simulink model "HVACRelay_harness"  (Simulink 7.7)
settings: Solver=FixedStepDiscrete  SolverMode=SingleTasking  StartTime=0.0  StopTime=100  FixedStep=.01  RelTol=1e-3
PostLoadFcn:
  | cd '..';
  | PostLoadFcn;
  | cd 'harness';
InitFcn:
  | if signalbuilder('HVACRelay_harness/Signal Builder','activegroup') == 1
  |   CD_HVAC_RELAY_FUNCTION.DataType = 'uint8';
  |   CD_HVAC_RELAY_FUNCTION.Value = 255;
  |   CD_HVAC_RELAY_FEEDBACK_FUNCTION.DataType = 'uint8';
  |   CD_HVAC_RELAY_FEEDBACK_FUNCTION.Value = 255;
  | else
  |   CD_HVAC_RELAY_FUNCTION.DataType = 'uint8';
  |   CD_HVAC_RELAY_FUNCTION.Value = 0;
  |   CD_HVAC_RELAY_FEEDBACK_FUNCTION.DataType = 'uint8';
  |   CD_HVAC_RELAY_FEEDBACK_FUNCTION.Value = 0;
  | end
undefined symbols (not defined in the file): ACTIVE, CD_HVAC_RELAY_DEBOUNCE_ERROR_ON, ENGINE_CRANKING, INACTIVE, NON_FUNCTIONAL, NORMAL, OORL, sigbuilder_block, srate, SYS_NORMAL
libraries: simulink x2, MX_Library x1
settings Model: Creator=smindema  LastModifiedBy=aliebel  CovMetricSettings=dcmw  CovHTMLOptions=-aTS=1 -bRG=1 -bTC=1 -hTR=0 -nFC=0 -scm=1 -bcm=1 -xEv=0  covSaveCumulativeToWorkspaceVar=off  CovSaveSingleToWorkspaceVar=off
settings MATStruct: SampleTime=0.01  Offset=0  Priority=[1.0]
settings DataIOCC: LimitDataPoints=off  SaveOutput=off  SaveTime=off
settings OptimizationCC: BlockReduction=off  InlineParams=on  ExpressionFolding=off  StateBitsets=on  DataBitsets=on  UseTempVars=on  InitFltsAndDblsToZero=on  NoFixptDivByZeroProtection=on  EfficientFloat2IntCast=on  OptimizeModelRefInitCode=on
settings DebuggingCC: SaveWithParameterizedLinksMsg=none  MultiTaskDSMMsg=warning  MultiTaskCondExecSysMsg=none  IntegerOverflowMsg=none  ModelReferenceCSMismatchMessage=warning
settings HardwareCC: ProdBitPerInt=16  ProdBitPerPointer=16  ProdIntDivRoundTo=Floor  ProdEndianess=BigEndian  ProdWordSize=16  ProdHWDeviceType=Motorola HC12
settings ModelReferenceCC: ModelReferenceNumInstancesAllowed=Single
settings RTWCC: SystemTargetFile=ert.tlc  GenCodeOnly=on  TemplateMakefile=ert_default_tmf  Description=Real-Time Workshop Embedded Coder (no auto configuration)  GenerateReport=on  RetainRTWFile=on  ProcessScript=ert_make_rtw_hook  IncludeHyperlinkInReport=on  LaunchReport=on  IncludeERTFirstTime=on
settings RTWCC: CustomHeaderCode=|
  | #include "cpp_req_defines.h"
  | #include "hw_fin.h"
  | #include "cdata.h"
settings CodeAppCC: IgnoreCustomStorageClasses=off  DefineNamingRule=UpperCase
settings ERTTargetCC: TargetFcnLib=ansi_tfl_tmw.mat  FunctionExecutionProfile=off  MultiwordLength=2048  GenerateSampleERTMain=on  IncludeMdlTerminateFcn=off  SupportAbsoluteTime=off  SupportNonFinite=off  SupportComplex=off  PurelyIntegerCode=on  ERTCustomFileTemplate=gen_rtw_req_defines_h.tlc  GlobalDataDefinition=InSeparateSourceFile  GlobalDataReference=InSeparateHeaderFile  ConvertIfToSwitch=off

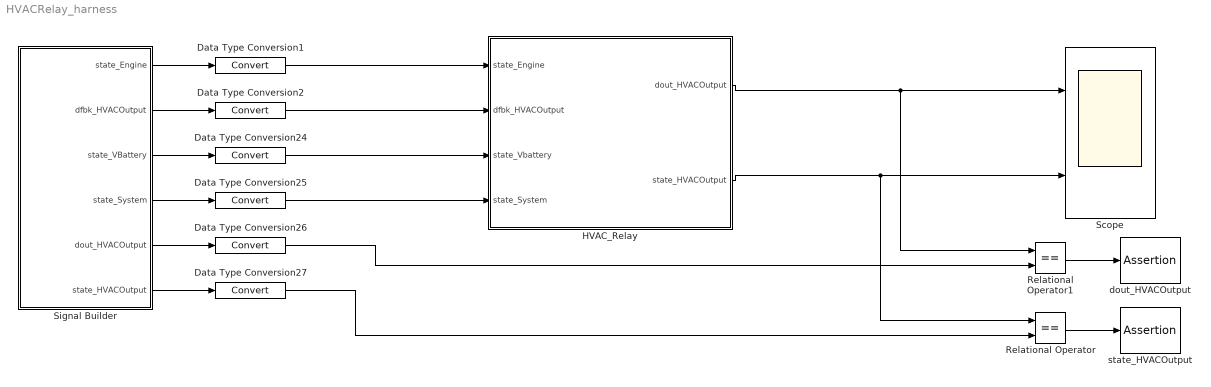
== system HVACRelay_harness ==
  Data Type Conversion{1..2,24..27} (6 alike) : DataTypeConversion
  HVAC_Relay : Subsystem  TreatAsAtomicUnit=on  SystemSampleTime=srate  RTWFileName=mod_Outputs
      settings: RTWSystemCode=Function  RTWFileNameOpts=User specified
  Relational Operator : RelationalOperator  Operator===  OutDataTypeStr=boolean
  Relational Operator1 : RelationalOperator  Operator===  OutDataTypeStr=boolean
  Scope : Scope  NumInputPorts=2
      settings: TimeRange=100  YMin=0~0  YMax=6~10  DataFormat=Array
  Signal Builder : Subsystem  Tag=STV Subsys  LoadFcn=sigbuilder_block('load');  StartFcn=sigbuilder_block('start');  StopFcn=sigbuilder_block('stop');  ClipboardFcn=sigbuilder_block('clipboard');  mask(Sigbuilder block){}
      mask help: Create and generate interchangeable groups of signals whose waveforms are piecewise linear.
      mask init:
      | if ~strcmp(get_param(bdroot(gcbh),'SimulationStatus'),'stopped') tuvar = sigbuilder_block('maskInit'); end
      settings: CopyFcn=sigbuilder_block('copy');  DeleteFcn=sigbuilder_block('delete');  ModelCloseFcn=sigbuilder_block('modelClose');  PreSaveFcn=sigbuilder_block('preSave');  NameChangeFcn=sigbuilder_block('namechange');  OpenFcn=sigbuilder_block('open',[1440 133.5 1440 753 ]);  CloseFcn=sigbuilder_block('close');
      mask Display: plot(0, 0, 100, 100,[2, 2, 32, 32, 2], [68, 8, 8, 68, 68],[32, 2], [38, 38], [32, 19, 2],[53, 60, 44], [32, 17, 17, 2],[16, 16, 31, 31]);txt = getActiveGroup(gcbh);text(2, 100, txt,'verticalAlignment', 'top');
  dout_HVACOutput : Assertion  Enabled=off
  state_HVACOutput : Assertion  Enabled=off
  wires:
  Relational Operator/1 -> state_HVACOutput/1
  Relational Operator1/1 -> dout_HVACOutput/1
  Data Type Conversion26/1 -> Relational Operator1/2
  Data Type Conversion27/1 -> Relational Operator/2
  HVAC_Relay/1(dout_HVACOutput) -> Scope/1, Relational Operator1/1
  HVAC_Relay/2(state_HVACOutput) -> Scope/2, Relational Operator/1
  Data Type Conversion2/1 -> HVAC_Relay/2(dfbk_HVACOutput)
  Data Type Conversion24/1 -> HVAC_Relay/3(state_Vbattery)
  Data Type Conversion25/1 -> HVAC_Relay/4(state_System)
  Signal Builder/1(state_Engine) -> Data Type Conversion1/1
  Signal Builder/2(dfbk_HVACOutput) -> Data Type Conversion2/1
  Signal Builder/5(dout_HVACOutput) -> Data Type Conversion26/1
  Signal Builder/6(state_HVACOutput) -> Data Type Conversion27/1
  Signal Builder/3(state_VBattery) -> Data Type Conversion24/1
  Signal Builder/4(state_System) -> Data Type Conversion25/1
  Data Type Conversion1/1 -> HVAC_Relay/1(state_Engine)

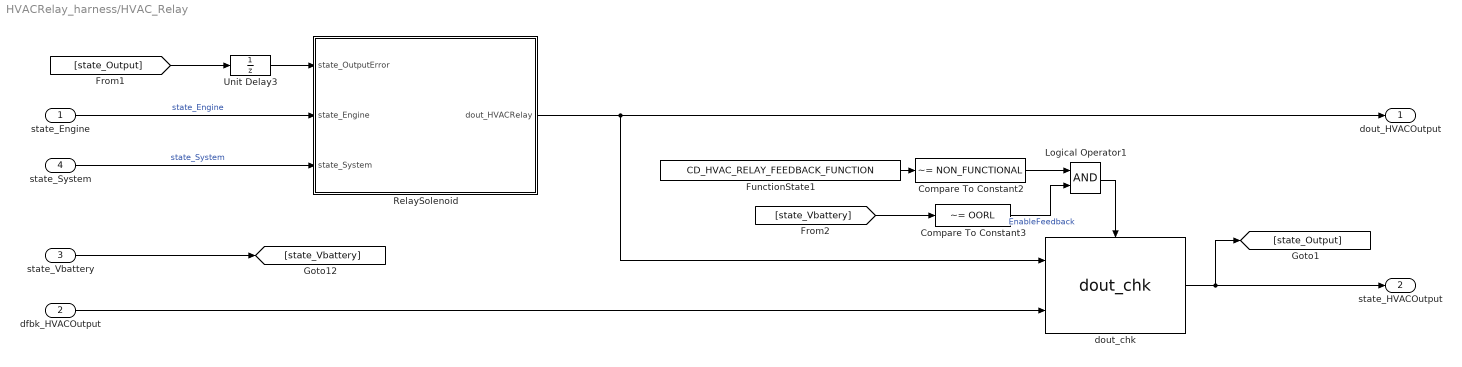
== system HVACRelay_harness/HVAC_Relay ==
  state_Engine : Inport  OutDataTypeStr=uint8
  dfbk_HVACOutput : Inport  Port=2
  state_Vbattery : Inport  Port=3
  state_System : Inport  Port=4  OutDataTypeStr=uint8
  Compare To Constant2 : simulink/Logic and Bit Operations/Compare To Constant  SystemSampleTime=-1  relop=~=  const=NON_FUNCTIONAL  LogicOutDataTypeMode=boolean  ZeroCross=off
  Compare To Constant3 : simulink/Logic and Bit Operations/Compare To Constant  SystemSampleTime=-1  relop=~=  const=OORL  LogicOutDataTypeMode=boolean  ZeroCross=off
  FunctionState1 : Constant  Value=CD_HVAC_RELAY_FEEDBACK_FUNCTION  OutDataTypeStr=uint8
  Logical Operator1 : Logic  AllPortsSameDT=off  OutDataTypeStr=boolean
  RelaySolenoid : Stateflow chart  TreatAsAtomicUnit=on
  Unit Delay3 : UnitDelay  SampleTime=-1
      settings: AttributesFormatString=<initial=%<X0>>\n<tsample=%<SampleTime>>
  dout_chk : MX_Library/dout_chk  SystemSampleTime=-1  ERR_ON_DB_CNT=CD_HVAC_RELAY_DEBOUNCE_ERROR_ON  ERR_OFF_DB_CNT=CD_HVAC_RELAY_DEBOUNCE_ERROR_OFF
  dout_HVACOutput : Outport  OutDataTypeStr=boolean
  state_HVACOutput : Outport  Port=2  OutDataTypeStr=uint8
  wires:
  RelaySolenoid/1(dout_HVACRelay) -> dout_HVACOutput/1, dout_chk/1
  dfbk_HVACOutput/1 -> dout_chk/2
  state_Engine/1 -> RelaySolenoid/2(state_Engine)  "state_Engine"
  state_System/1 -> RelaySolenoid/3(state_System)  "state_System"
  state_Vbattery/1 -> [state_Vbattery]
  dout_chk/1 -> [state_Output], state_HVACOutput/1
  Compare To Constant3/1 -> Logical Operator1/2  "EnableFeedback"
  Logical Operator1/1 -> dout_chk/Enable
  FunctionState1/1 -> Compare To Constant2/1
  Compare To Constant2/1 -> Logical Operator1/1
  Unit Delay3/1 -> RelaySolenoid/1(state_OutputError)
  [state_Output] -> Unit Delay3/1
  [state_Vbattery] -> Compare To Constant3/1

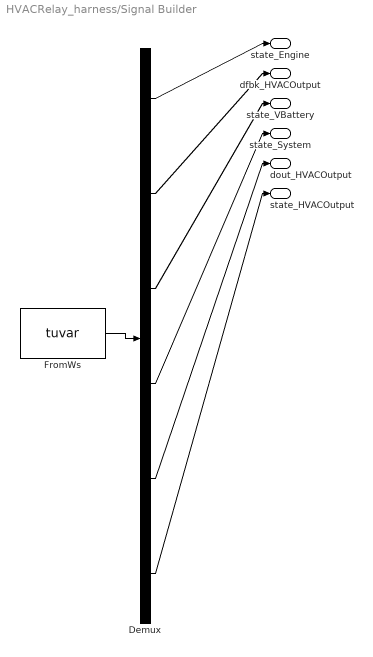
== system HVACRelay_harness/Signal Builder ==
  Demux : Demux  Tag=STV Demux  Outputs=6
  FromWs : FromWorkspace  Tag=STV FromWs  VariableName=tuvar  SampleTime=0  SigBuilderData=DataTag0  VnvData=DataTag1
      SigBuilderData=|
      | common.afterFinalStr = 'Extrapolate'
      | common.sampleTime = 0
      | dataSet(1).timeRange = [0 100]
      | dataSet(1).name = 'NonFunctional'
      | dataSet(2).timeRange = [0 100]
      | dataSet(2).name = 'Functional1'
      | sbobj.Groups(1).Name = 'NonFunctional'
      | sbobj.Groups(1).Signals(1).Name = 'state_Engine'
      | sbobj.Groups(1).Signals(1).XData = [0 2 2 4 4 6 6 8 8 10 10 12 12 14 14 16 16 18 18 20 20 22 22 24 24 26 37 41 45 50 56 60 63 100]
      | sbobj.Groups(1).Signals(1).YData = [1 1 2 2 1 1 2 2 1 1 2 2 1 1 2 2 1 1 2 2 1 1 2 2 1 1 1 1 1 1 1 1 1 1]
      | sbobj.Groups(1).Signals(2).Name = 'dfbk_HVACOutput'
      | sbobj.Groups(1).Signals(2).XData = [0 6 6 12 12 18 18 24 24 30 59.8 66 75.5 100]
      | sbobj.Groups(1).Signals(2).YData = [0 0 1 1 0 0 1 1 0 0 0 0 0 0]
      | sbobj.Groups(1).Signals(3).Name = 'state_VBattery'
      | sbobj.Groups(1).Signals(3).XData = [0 100]
      | sbobj.Groups(1).Signals(3).YData = [8 8]
      | sbobj.Groups(1).Signals(4).Name = 'state_System'
      | sbobj.Groups(1).Signals(4).XData = [0 12 12 24 24 48 56 100]
      | sbobj.Groups(1).Signals(4).YData = [1 1 5 5 1 1 1 1]
      | sbobj.Groups(1).Signals(5).Name = 'dout_HVACOutput'
      | sbobj.Groups(1).Signals(5).XData = [0 100]
      | sbobj.Groups(1).Signals(5).YData = [0 0]
      | sbobj.Groups(1).Signals(6).Name = 'state_HVACOutput'
      | sbobj.Groups(1).Signals(6).XData = [0 100]
      | sbobj.Groups(1).Signals(6).YData = [8 8]
      | sbobj.Groups(1).TimeRange = [0 100]
      | sbobj.Groups(2).Name = 'Functional1'
      | sbobj.Groups(2).Signals(1).Name = 'state_Engine'
      | sbobj.Groups(2).Signals(1).XData = [0 13 13 15 15 24 27 41.03 41.03 45 45 100]
      | sbobj.Groups(2).Signals(1).YData = [1 1 2 2 1 1 1 1 2 2 1 1]
      | sbobj.Groups(2).Signals(2).Name = 'dfbk_HVACOutput'
      | sbobj.Groups(2).Signals(2).XData = [0 0.38 0.38 5.01 5.01 11.01 11.01 13.01 13.01 15.01 15.01 18.01 18.01 20.1 20.1 25.03 25.03 41.03 41.03 75.5 100]
      | sbobj.Groups(2).Signals(2).YData = [0 0 1 1 0 0 1 1 0 0 1 1 0 0 1 1 0 0 1 1 1]
      | sbobj.Groups(2).Signals(3).Name = 'state_VBattery'
      | sbobj.Groups(2).Signals(3).XData = [0 10 10 11 11 25 25 26 26 40 40 41 41 100]
      | sbobj.Groups(2).Signals(3).YData = [8 8 22 22 8 8 22 22 8 8 22 22 8 8]
      | sbobj.Groups(2).Signals(4).Name = 'state_System'
      | sbobj.Groups(2).Signals(4).XData = [0 18 18 23 23 48 56 100]
      | sbobj.Groups(2).Signals(4).YData = [1 1 5 5 1 1 1 1]
      | sbobj.Groups(2).Signals(5).Name = 'dout_HVACOutput'
      | sbobj.Groups(2).Signals(5).XData = [0 10.01 10.01 13 13 15 15 18 18 25.01 25.01 26.06 26.06 40.01 40.01 41.03 41.03 100]
      | sbobj.Groups(2).Signals(5).YData = [0 0 1 1 0 0 1 1 0 0 1 1 0 0 1 1 0 0]
      | sbobj.Groups(2).Signals(6).Name = 'state_HVACOutput'
      | sbobj.Groups(2).Signals(6).XData = [0 0.88 0.88 10 10 20.6 20.6 25 25 26.05 26.05 40 40 41.53 41.53 100]
      | sbobj.Groups(2).Signals(6).YData = [8 8 2 2 8 8 2 2 8 8 3 3 8 8 2 2]
      | sbobj.Groups(2).TimeRange = [0 100]
  state_Engine : Outport  Tag=STV Outport
  dfbk_HVACOutput : Outport  Tag=STV Outport  Port=2
  state_VBattery : Outport  Tag=STV Outport  Port=3
  state_System : Outport  Tag=STV Outport  Port=4
  dout_HVACOutput : Outport  Tag=STV Outport  Port=5
  state_HVACOutput : Outport  Tag=STV Outport  Port=6
  wires:
  FromWs/1 -> Demux/1
  Demux/1 -> state_Engine/1
  Demux/2 -> dfbk_HVACOutput/1
  Demux/3 -> state_VBattery/1
  Demux/4 -> state_System/1
  Demux/5 -> dout_HVACOutput/1
  Demux/6 -> state_HVACOutput/1

== stateflow chart HVAC_Relay/RelaySolenoid ==
  state INACTIVE
    en:dout_HVACRelay = INACTIVE;
  state ACTIVE
    en:dout_HVACRelay = ACTIVE;
  state STARTUP_ERROR_ON_CHECK
    en:dout_HVACRelay = INACTIVE;
    en:debounceCount = 0;
    du:debounceCount++;
  INACTIVE -> ACTIVE : [(CD_HVAC_RELAY_FUNCTION != NON_FUNCTIONAL)...
      | && (state_Engine != ENGINE_CRANKING)...
      | && (state_OutputError == NORMAL)...
      | && (state_System == SYS_NORMAL)]
  (default) -> STARTUP_ERROR_ON_CHECK
  ACTIVE -> INACTIVE : [(state_Engine == ENGINE_CRANKING)...
      | || (state_OutputError != NORMAL)...
      | || (state_System != SYS_NORMAL)]
  STARTUP_ERROR_ON_CHECK -> INACTIVE : [(debounceCount >= CD_HVAC_RELAY_DEBOUNCE_ERROR_ON + 100)]
  data: dout_HVACRelay output boolean; state_OutputError input uint8; state_Engine input uint8; ACTIVE parameter uint8 =1; ENGINE_CRANKING parameter uint8 =2; INACTIVE parameter uint8 =1; NORMAL parameter uint8 =1; NON_FUNCTIONAL parameter uint8; CD_HVAC_RELAY_FUNCTION parameter uint8; state_System input uint8; SYS_NORMAL parameter uint8; debounceCount local uint16; CD_HVAC_RELAY_DEBOUNCE_ERROR_ON parameter uint16
